simulink model "CVS_LVAD_2021a"  (R2021a)
settings: Solver=ode4  StartTime=0.0  StopTime=end_t  FixedStep=dt_step  RelTol=1e-3
values from neighbouring files (symbols this model uses):
  Cac = 13.7054    [SimMDL_Parameters.m]
  Cbc = 0.25    [SimMDL_Parameters.m]
  Cpa = 1/1.27    (= 0.787401574803)    [SimMDL_Parameters.m]
  Cpv = 1/0.247    (= 4.04858299595)    [SimMDL_Parameters.m]
  Csae = 1/3.02    (= 0.331125827815)    [SimMDL_Parameters.m]
  Csai = 1/7.76    (= 0.128865979381)    [SimMDL_Parameters.m]
  Csve = 1/0.0918    (= 10.8932461874)    [SimMDL_Parameters.m]
  Csvi = 1/0.0989    (= 10.111223458)    [SimMDL_Parameters.m]
  Da0 = 0    [SimMDL_Parameters.m]
  de_gain = 1.5    [SimMDL_Parameters.m]
  delay = 0.5*Tc    (= 0.230769230769)    [SimMDL_Parameters.m]
  deltastar = 0.5    [SimMDL_Parameters.m]
  DElv = 2*(Tc/0.833)    (= 1.10813556192)    [SimMDL_Parameters.m]
  DErv = 2*(Tc/0.833)    (= 1.10813556192)    [SimMDL_Parameters.m]
  Dm0 = 1    [SimMDL_Parameters.m]
  Dp0 = 0    [SimMDL_Parameters.m]
  DRsp = 3*(Tc/0.833)    (= 1.66220334288)    [SimMDL_Parameters.m]
  Dt0 = 1    [SimMDL_Parameters.m]
  dt_step = 1e-3    (= 0.001)    [SimMDL_Parameters.m]
  DTs = 3*(Tc/0.833)    (= 1.66220334288)    [SimMDL_Parameters.m]
  DTv = 0.5    [SimMDL_Parameters.m]
  e_gain = 2    [SimMDL_Parameters.m]
  Elamax = 1.99    [SimMDL_Parameters.m]
  Elamin = 0.733    [SimMDL_Parameters.m]
  Elvmax = 28.4    [SimMDL_Parameters.m]
  Elvmin = 0.550    (= 0.55)    [SimMDL_Parameters.m]
  Eramax = 0.63    [SimMDL_Parameters.m]
  Eramin = 0.317    [SimMDL_Parameters.m]
  Erv_max_sat = 1.2*Ervmax    (= 2.508)    [SimMDL_Parameters.m]
  Erv_max_thres = 0.8*Ervmax    (= 1.672)    [SimMDL_Parameters.m]
  Ervmax = 2.09    [SimMDL_Parameters.m]
  Ervmin = 0.348    [SimMDL_Parameters.m]
  Ga_Elv = 0.012    [SimMDL_Parameters.m]
  Ga_Erv = 0.012    [SimMDL_Parameters.m]
  Ga_Rsp = 0.1    [SimMDL_Parameters.m]
  GaTs = 0.015    [SimMDL_Parameters.m]
  GaTv = 0.028    [SimMDL_Parameters.m]
  Gp_Elv = 0    [SimMDL_Parameters.m]
  Gp_Erv = 0    [SimMDL_Parameters.m]
  Gp_Rsp = 0.33    [SimMDL_Parameters.m]
  GpTs = 0    [SimMDL_Parameters.m]
  GpTv = 0.25    [SimMDL_Parameters.m]
  k_Elv = (Elv_max_sat-Elv_max_thres)/(4*SElvo)    (= 2.84)    [SimMDL_Parameters.m]
  k_Erv = (Erv_max_sat-Erv_max_thres)/(4*SErvo)    (= 0.209)    [SimMDL_Parameters.m]
  k_Rsp = (Rsp_max-Rsp_min)/(4*SRspo)    (= 0.375)    [SimMDL_Parameters.m]
  Kn = max(Kn)    [SimMDL_Parameters.m]
  kT = (T_max-T_min)/(4*STo)    (= 0.035)    [SimMDL_Parameters.m]
  Li = 0.0402    [SimMDL_Parameters.m]
  Lo = 0.0426    [SimMDL_Parameters.m]
  Lsae = 0.0002    [SimMDL_Parameters.m]
  n = length(T)    [SimMDL_Parameters.m]
  pac0 = 0    [SimMDL_Parameters.m]
  pbc0 = 0    [SimMDL_Parameters.m]
  ppa0 = 8.5    [SimMDL_Parameters.m]
  ppv0 = 8    [SimMDL_Parameters.m]
  psae0 = 70    [SimMDL_Parameters.m]
  psai0 = 75    [SimMDL_Parameters.m]
  Psan = 75    [SimMDL_Parameters.m]
  psve0 = 8.7    [SimMDL_Parameters.m]
  psvi0 = 6    [SimMDL_Parameters.m]
  Pth = -3.25    [SimMDL_Parameters.m]
  qi0 = 0    [SimMDL_Parameters.m]
  qo0 = 0    [SimMDL_Parameters.m]
  qsae0 = 10    [SimMDL_Parameters.m]
  Rac = 0.0025    [SimMDL_Parameters.m]
  Ri = 0.4283    [SimMDL_Parameters.m]
  Rm = 0.006    [SimMDL_Parameters.m]
  Ro = 1.2841    [SimMDL_Parameters.m]
  Rpa = 0.006    [SimMDL_Parameters.m]
  Rpp = 0.220    (= 0.22)    [SimMDL_Parameters.m]
  Rpv = 0.006    [SimMDL_Parameters.m]
  Rsae = 0.120    (= 0.12)    [SimMDL_Parameters.m]
  Rsai = 0.016    [SimMDL_Parameters.m]
  Rsp = 2.00    (= 2)    [SimMDL_Parameters.m]
  Rsp_max = 3    [SimMDL_Parameters.m]
  Rsp_min = 1.5    [SimMDL_Parameters.m]
  Rsve = 0.18    [SimMDL_Parameters.m]
  Rsvi = 0.006    [SimMDL_Parameters.m]
  Rtv = 0.006    [SimMDL_Parameters.m]
  t_eject = (Tc*ts_VAD)/dt_step    (= 230.769230769)    [SimMDL_Parameters.m]
  T_max = 0.535    [SimMDL_Parameters.m]
  T_min = 0.395    [SimMDL_Parameters.m]
  Tas = 0.03+0.09*Tc    (= 0.0715384615385)    [SimMDL_Parameters.m]
  Tau_Elv = 1.5    [SimMDL_Parameters.m]
  Tau_Erv = 1.5    [SimMDL_Parameters.m]
  Tau_Rsp = 1.5    [SimMDL_Parameters.m]
  Tau_Ts = 1.8    [SimMDL_Parameters.m]
  Tau_Tv = 0.8    [SimMDL_Parameters.m]
  Tav = 0.01    [SimMDL_Parameters.m]
  Tc = 60/HR    (= 0.461538461538)    [SimMDL_Parameters.m]
  ts_VAD = 0.5    [SimMDL_Parameters.m]
  tune_alpha = x(5)    [SimMDL_Parameters.m]
  tune_gamma = x(3)    [SimMDL_Parameters.m]
  tune_lambda1 = x(1)    [SimMDL_Parameters.m]
  tune_lambda2 = x(2)    [SimMDL_Parameters.m]
  tune_nu = x(4)    [SimMDL_Parameters.m]
  Tvs = 0.16+0.20*Tc    (= 0.252307692308)    [SimMDL_Parameters.m]
  VAD_delay = ts_VAD    (= 0.5)    [SimMDL_Parameters.m]
  vla0 = 11.2524    [SimMDL_Parameters.m]
  Vlau = 1.0    (= 1)    [SimMDL_Parameters.m]
  Vln = 2.3    [SimMDL_Parameters.m]
  vlv0 = 15.6126    [SimMDL_Parameters.m]
  Vlvu = 2.0    (= 2)    [SimMDL_Parameters.m]
  vra0 = 22.36    [SimMDL_Parameters.m]
  Vrau = 1.5    [SimMDL_Parameters.m]
  vrv0 = 26.99    [SimMDL_Parameters.m]
  Vrvu = 3.0    (= 3)    [SimMDL_Parameters.m]
undefined symbols (not defined in the file or in its folder): D_E_max_lv, D_E_max_rv, D_R_svr, D_Ts, D_Tv, f_as_0, f_es_0, f_es_inf, f_es_min, f_ev_0, f_ev_inf, f_max, f_min, G_E_max_lv, G_E_max_rv, G_R_svr, G_Ts, G_Tv, HP_gain, HP_max, HP_min, HP_op, k_es, k_ev, ka, mPsai_op, mPsai_sat, mPsai_thres, passo, pn, Tau_E_max_lv, Tau_E_max_rv, Tau_p, Tau_R_svr, Tau_z
libraries: simulink x6, spsSampleandHoldLib x5, dspmathops x1
(part 2 of 2)

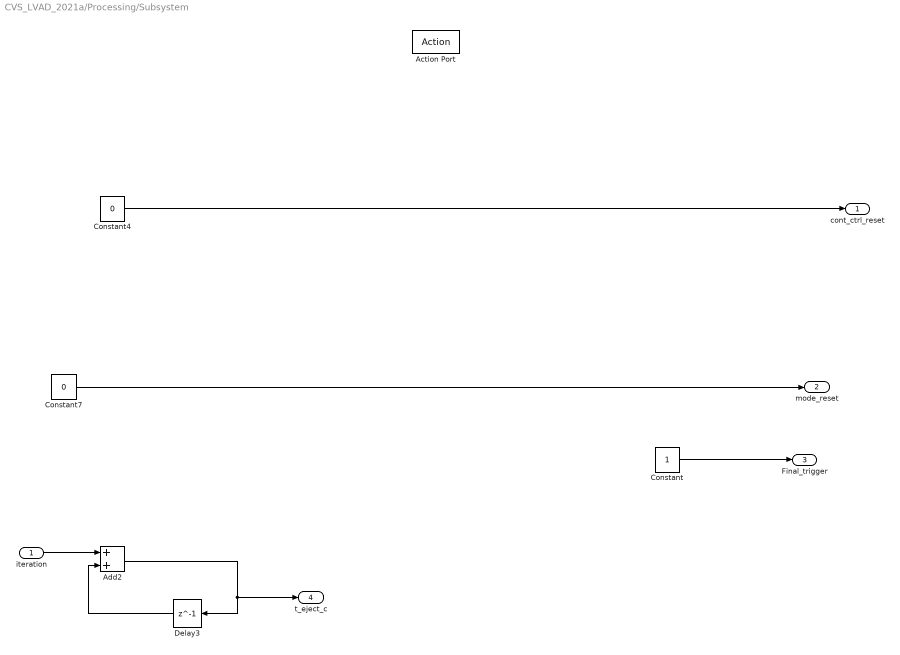
== system CVS_LVAD_2021a/Processing/Subsystem ==
  iteration : Inport
  Action Port : ActionPort  ActionPortLabel=if(u1 > u2)
  Add2 : Sum
  Constant : Constant
  Constant4 : Constant  Value=0
  Constant7 : Constant  Value=0
  Delay3 : Delay  DelayLength=1
  cont_ctrl_reset : Outport
  mode_reset : Outport  Port=2
  Final_trigger : Outport  Port=3
  t_eject_c : Outport  Port=4
  wires:
  Delay3/1 -> Add2/2
  iteration/1 -> Add2/1
  Add2/1 -> t_eject_c/1, Delay3/1
  Constant4/1 -> cont_ctrl_reset/1
  Constant7/1 -> mode_reset/1
  Constant/1 -> Final_trigger/1

== system CVS_LVAD_2021a/Processing/Subsystem1 ==
  Action Port : ActionPort  ActionPortLabel=else
  Constant : Constant  Value=0
  Constant5 : Constant
  Constant8 : Constant
  Cont_ctrl_copy : Outport
  mode_copy : Outport  Port=2
  Final_trigger : Outport  Port=3
  wires:
  Constant8/1 -> mode_copy/1
  Constant5/1 -> Cont_ctrl_copy/1
  Constant/1 -> Final_trigger/1

== system CVS_LVAD_2021a/Processing/Subsystem2 ==
  mode : Inport
  iteration : Inport  Port=2
  t_eject_c : Inport  Port=3
  Action Port : ActionPort  ActionPortLabel=else
  If Action Subsystem : Subsystem  TreatAsAtomicUnit=on
  If2 : If  NumInputs=3  IfExpression=u1 == 1 & u2>=u2  ShowElse=off
  reset : Constant  Value=0
  Out1 : Outport
  Pd_fill : Outport  Port=2
  wires:
  reset/1 -> If Action Subsystem/2(mode_update), If Action Subsystem/1(Pd_fill)
  If2/1 -> If Action Subsystem/Action
  If Action Subsystem/1(Out1) -> Pd_fill/1
  t_eject_c/1 -> If2/3
  mode/1 -> If2/1
  If Action Subsystem/2(Out2) -> Out1/1
  iteration/1 -> If2/2

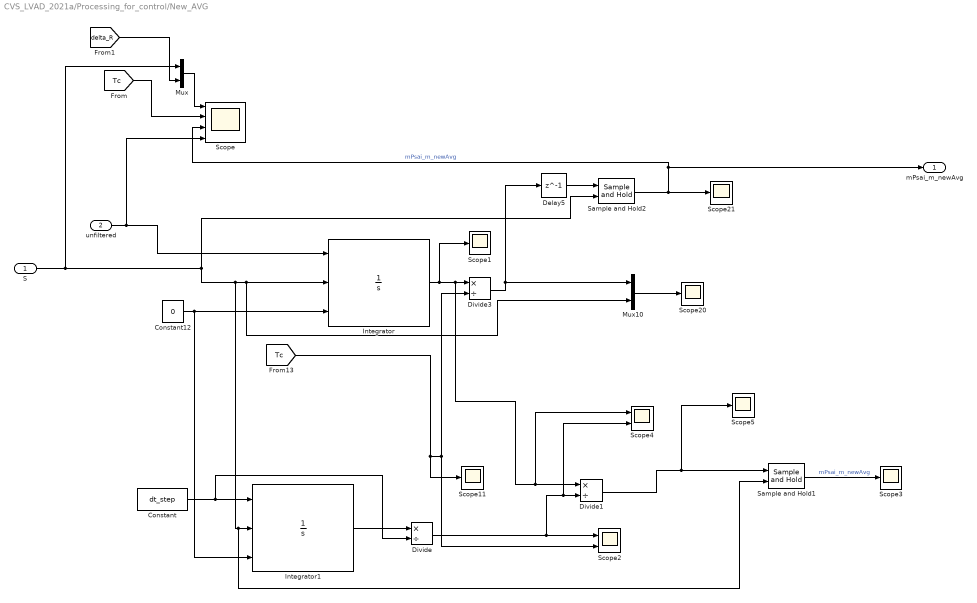
== system CVS_LVAD_2021a/Processing_for_control/New_AVG ==
  S : Inport
  unfiltered : Inport  Port=2
  Constant : Constant  Value=dt_step
  Constant12 : Constant  Value=0
  Delay5 : Delay  DelayLength=1  InitialCondition=psai0
  Divide : Product  Inputs=*/
  Divide1 : Product  Inputs=*/
  Divide3 : Product  Inputs=*/
  Integrator : Integrator  ExternalReset=rising  InitialConditionSource=external
  Integrator1 : Integrator  ExternalReset=rising  InitialConditionSource=external
  Mux : Mux  Inputs=2
  Mux10 : Mux  Inputs=2
  Sample and Hold1 : spsSampleandHoldLib/Sample and Hold  ic=psai0  Ts=dt_step
      settings: SourceProductBaseCode=PS
  Sample and Hold2 : spsSampleandHoldLib/Sample and Hold  ic=psai0  Ts=dt_step
      settings: SourceProductBaseCode=PS
  Scope : Scope  NumInputPorts=4
  Scope{1,3,5,11,20..21} (6 alike) : Scope
  Scope2 : Scope  NumInputPorts=2
  Scope4 : Scope  NumInputPorts=2
  mPsai_m_newAvg : Outport
  wires:
  [Tc] -> Scope2/2, Divide3/2, Scope11/1
  Sample and Hold2/1 -> mPsai_m_newAvg/1, Scope/3, Scope21/1  "mPsai_m_newAvg"
  unfiltered/1 -> Scope/4, Integrator/1
  Delay5/1 -> Sample and Hold2/1
  Mux10/1 -> Scope20/1
  Divide3/1 -> Delay5/1, Mux10/1
  Integrator/1 -> Scope1/1, Scope4/1, Divide1/1, Divide3/1
  Constant12/1 -> Integrator/3, Integrator1/3
  [Tc] -> Scope/2
  [delta_R] -> Mux/2
  Mux/1 -> Scope/1
  Constant/1 -> Divide/2, Integrator1/1
  Integrator1/1 -> Divide/1
  Divide/1 -> Scope4/2, Divide1/2, Scope2/1
  Sample and Hold1/1 -> Scope3/1  "mPsai_m_newAvg"
  Divide1/1 -> Scope5/1, Sample and Hold1/1
  S/1 -> Mux/1, Integrator/2, Mux10/2, Sample and Hold1/2, Integrator1/2, Sample and Hold2/2

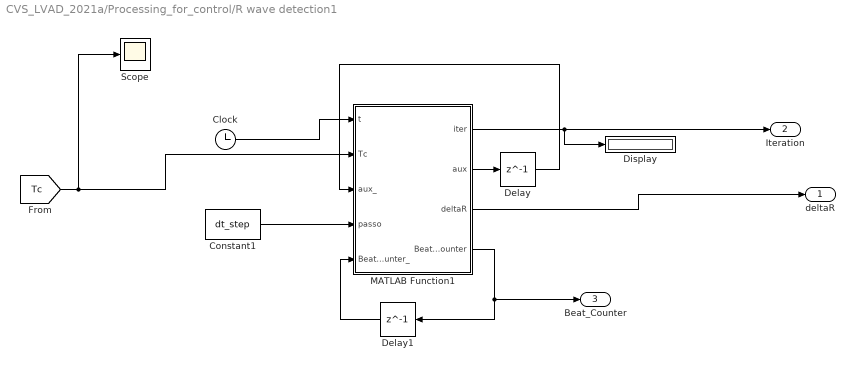
== system CVS_LVAD_2021a/Processing_for_control/R wave detection1 ==
  Clock : Clock
  Constant1 : Constant  Value=dt_step
  Delay : Delay  DelayLength=1
  Delay1 : Delay  DelayLength=1  InitialCondition=0
  Display : Display
  MATLAB Function1 : MATLAB Function  TreatAsAtomicUnit=on
  Scope : Scope
  deltaR : Outport
  Iteration : Outport  Port=2
  Beat_Counter : Outport  Port=3
  wires:
  MATLAB Function1/2(aux) -> Delay/1
  MATLAB Function1/1(iter) -> Display/1, Iteration/1
  Clock/1 -> MATLAB Function1/1(t)
  Constant1/1 -> MATLAB Function1/4(passo)
  MATLAB Function1/3(deltaR) -> deltaR/1
  Delay/1 -> MATLAB Function1/3(aux_)
  MATLAB Function1/4(Beat_Counter) -> Beat_Counter/1, Delay1/1
  Delay1/1 -> MATLAB Function1/5(Beat_Counter_)
  [Tc] -> Scope/1, MATLAB Function1/2(Tc)

== system CVS_LVAD_2021a/Processing_for_control/Subsystem ==
  e(n) : Inport
  e(n-1) : Inport  Port=2
  Gain3 : Gain  Gain=1/dt_step
  Subtract : Sum  Inputs=+-
  de/dt : Outport
  wires:
  Subtract/1 -> Gain3/1
  Gain3/1 -> de/dt/1
  e(n)/1 -> Subtract/1
  e(n-1)/1 -> Subtract/2

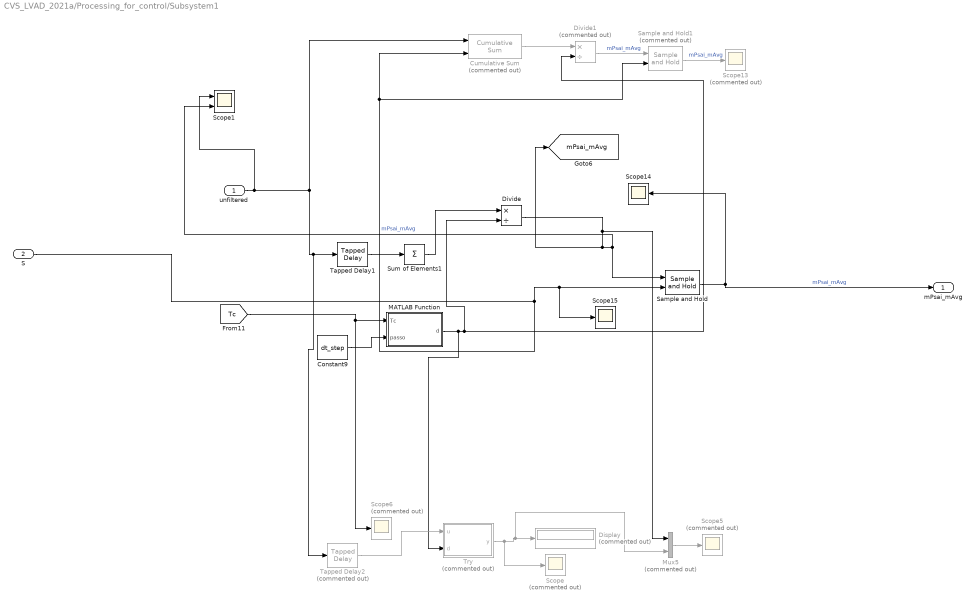
== system CVS_LVAD_2021a/Processing_for_control/Subsystem1 ==
  unfiltered : Inport
  S : Inport  Port=2
  Constant9 : Constant  Value=dt_step
  Cumulative Sum : dspmathops/Cumulative Sum  Commented=on  dim=Channels (running sum)  reset_popup=Non-zero sample  roundingMode=Floor  overflowMode=off  outputDataTypeStr=Inherit: Same as accumulator  outputMin=[]  outputMax=[]  outputLastDataTypeStr=Inherit: Same as accumulator
  Display : Display  Commented=on
  Divide : Product  Inputs=*/
  Divide1 : Product  Commented=on  Inputs=*/
  MATLAB Function : MATLAB Function  TreatAsAtomicUnit=on
  Mux5 : Mux  Commented=on  Inputs=2
  Sample and Hold : spsSampleandHoldLib/Sample and Hold  ic=psai0  Ts=dt_step
      settings: SourceProductBaseCode=PS
  Sample and Hold1 : spsSampleandHoldLib/Sample and Hold  Commented=on  ic=psai0  Ts=passo
      settings: SourceProductBaseCode=PS
  Scope{,5..6,13} (4 alike) : Scope  Commented=on
  Scope1 : Scope  NumInputPorts=2
  Scope14 : Scope
  Scope15 : Scope
  Sum of Elements1 : Sum  Inputs=+
  Tapped Delay1 : simulink/Discrete/Tapped Delay  vinit=psai0  samptime=-1  NumDelays=ceil(Tc/dt_step)  DelayOrder=Oldest  includeCurrent=on
  Tapped Delay2 : simulink/Discrete/Tapped Delay  Commented=on  vinit=psai0  samptime=-1  NumDelays=6000  DelayOrder=Oldest  includeCurrent=on
  Try : MATLAB Function  Commented=on  TreatAsAtomicUnit=on
  mPsai_mAvg : Outport
  tag scope: mPsai_mAvg=global
  wires:
  Sum of Elements1/1 -> Divide/1
  MATLAB Function/1(d) -> Divide1/2, Divide/2, Try/2(d)
  S/1 -> Sample and Hold/2, Scope15/1, Sample and Hold1/2, Cumulative Sum/2
  [Tc] -> MATLAB Function/1(Tc), Scope6/1
  Constant9/1 -> MATLAB Function/2(passo)
  Mux5/1 -> Scope5/1
  unfiltered/1 -> Scope1/1, Tapped Delay2/1, Tapped Delay1/1, Cumulative Sum/1
  Try/1(y) -> Scope/1, Mux5/2, Display/1
  Divide/1 -> Mux5/1, [mPsai_mAvg], Scope1/2, Sample and Hold/1  "mPsai_mAvg"
  Tapped Delay1/1 -> Sum of Elements1/1
  Tapped Delay2/1 -> Try/1(u)
  Sample and Hold/1 -> mPsai_mAvg/1, Scope14/1  "mPsai_mAvg"
  Divide1/1 -> Sample and Hold1/1  "mPsai_mAvg"
  Sample and Hold1/1 -> Scope13/1  "mPsai_mAvg"
  Cumulative Sum/1 -> Divide1/1

== system CVS_LVAD_2021a/Processing/Subsystem2/If Action Subsystem ==
  Pd_fill : Inport
  mode_update : Inport  Port=2
  Action Port : ActionPort  ActionPortLabel=if(u1 == 1 & u2>=u2)
  Out1 : Outport
  Out2 : Outport  Port=2
  wires:
  Pd_fill/1 -> Out1/1
  mode_update/1 -> Out2/1

== matlab function CVS_LVAD_2021a/Baroreflex Model_Liu/MATLAB Function3 ==
  data: G_E_max_rv input; sigma_E_max_rv output; f_es_min input; f_es input
function sigma_E_max_rv = fcn(G_E_max_rv,f_es_min,f_es)

if(f_es>=f_es_min)
    sigma_E_max_rv = G_E_max_rv*log(f_es-f_es_min+1);
else
    sigma_E_max_rv = 0;
end

== matlab function CVS_LVAD_2021a/Baroreflex Model_Liu/MATLAB Function4 ==
  data: G_Ts input; sigma_Ts output; f_es_min input; f_es input
function sigma_Ts = fcn(G_Ts,f_es_min,f_es)

if(f_es>=f_es_min)
    sigma_Ts = G_Ts*log(f_es-f_es_min+1);
else
    sigma_Ts = 0;
end

== matlab function CVS_LVAD_2021a/Heart+LVAD1/MATLAB Function ==
  data: Tas input; Kn output; Tav input; Tvs input; Tc input; n input; iter input
function Kn = fcn(Tas,Tav,Tvs,Tc,n,iter)
Kn_=zeros(1,n);
for k = 1:n
   j = mod(iter, Tc);
   Kn_(k) = ((j-(Tas + Tav))/Tvs)*sin((pi*(j-(Tas + Tav))/Tvs));
end
Kn = max(Kn_);

== matlab function CVS_LVAD_2021a/Controller/MATLAB Function1 ==
  data: PID input; u output; Dual input; SM input; sw input
function u = fcn(PID,Dual,SM,sw)

if(sw==0)
    u=PID;
elseif(sw==1)
    u=SM;
else
    u=Dual;
end

== matlab function CVS_LVAD_2021a/Processing_for_control/Subsystem1/MATLAB Function ==
  data: Tc input; d output; passo input
function d = fcn(Tc,passo)
%#codegen
d=(ceil(Tc/passo));

== matlab function CVS_LVAD_2021a/Processing_for_control/Subsystem1/Try ==
  data: u input; y output; d input
function y = fcn(u,d)

sum=0;
for i= (5000-d+1):5000
    sum=sum+u(i);
end
y=sum/d;

== matlab function CVS_LVAD_2021a/Ursino Model/MATLAB Function1 ==
  data: t input; HP output; HP_baro input; HP_Prev input
function HP = fcn(t,HP_baro,HP_Prev)

if(t>0)
    if(mod(t,5)==0)
        HP=HP_baro;
    else
        HP=HP_Prev;
    end
else
    HP=HP_Prev;
end

== matlab function CVS_LVAD_2021a/Controller/Cordeiro's _Controller ==
  data: Pe_n_1 input; Pe output; Pe_n_2 input; Pe_n_3 input; e_n input; e_n_1 input; e_n_2 input; e_n_3 input
function Pe = fcn(Pe_n_1,Pe_n_2, Pe_n_3,e_n, e_n_1,  e_n_2, e_n_3)

num = [1.0000    2.3082   -0.1752    0.0017];
b0 =  num(1);
b1 =  num(2);
b2 =  num(3);
b3 =  num(4);

den = [1.0000   -0.4633   -0.9876    0.4509];
a0 =  den(1);
a1 =  den(2);
a2 =  den(3);
a3 =  den(4);
%Pe = (-a1/a0)*Pe(ii-1) + (-a2/a0)*Pe(ii-2) + (-a3/a0)*Pe(ii-3)...
                         %  + (b0/a0)*e(ii) + (b1/a0)*e(ii-1) + (b2/a0)*e(ii-2) + (b3/a0)*e(ii-3);
Pe = (-a1/a0)*Pe_n_1 + (-a2/a0)*Pe_n_2 + (-a3/a0)*Pe_n_3 + (b0/a0)*e_n + (b1/a0)*e_n_1 + (b2/a0)*e_n_2 + (b3/a0)*e_n_3;

== matlab function CVS_LVAD_2021a/Processing_for_control/Fig7_Cordeiro2020 ==
  data: Beats_c input; mPsai_ref output
function mPsai_ref = fcn(Beats_c)

mPsai_ref=75;
if (Beats_c >= 25) && (Beats_c < 70)
    mPsai_ref = 85;
elseif (Beats_c >=70)
    mPsai_ref = 80;

end

== matlab function CVS_LVAD_2021a/Ursino Model/Sigmoid_Rsp ==
  data: Rsp_min input; sigma_Rsp output; Rsp_max input; k_Rsp input; x_Rsp input
function sigma_Rsp = fcn(Rsp_min,Rsp_max,k_Rsp,x_Rsp)


num=Rsp_min+Rsp_max*exp(-x_Rsp/k_Rsp);
den=1+exp(-x_Rsp/k_Rsp);
sigma_Rsp = num/den;

== matlab function CVS_LVAD_2021a/Ursino Model/Sigmoid_T ==
  data: T_min input; T output; T_max input; kT input; xT input
function T = fcn(T_min,T_max,kT,xT)

num=T_min+T_max*exp(xT/kT);
den=1+exp(xT/kT);
T=num/den;

== matlab function CVS_LVAD_2021a/Ursino Model/Sigmoid_Rsp1 ==
  data: Erv_min input; sigma_Erv output; Erv_max input; k_Erv input; x_Erv input
function sigma_Erv = fcn(Erv_min,Erv_max,k_Erv,x_Erv)


num=Erv_min+Erv_max*exp(-x_Erv/k_Erv);
den=1+exp(-x_Erv/k_Erv);
sigma_Erv = num/den;

== matlab function CVS_LVAD_2021a/Ursino Model/MATLAB Function ==
  data: Y_min input; Y output; Y_max input; X_thres input; X_sat input; X0 input; Y0 input; X input; gain input
function Y = fcn(Y_min,Y_max,X_thres,X_sat,X0,Y0,X,gain)

%X0 and Y0 are redundant
if(X<=X_thres)
    Y=Y_min;
elseif(X>=X_sat)
    Y=Y_max;
else
    Y=Y0+gain*(X-X0);
end

== matlab function CVS_LVAD_2021a/Ursino Model/Sigmoid_Rsp2 ==
  data: Elv_min input; sigma_Elv output; Elv_max input; k_Elv input; x_Elv input
function sigma_Elv = fcn(Elv_min,Elv_max,k_Elv,x_Elv)


num=Elv_min+Elv_max*exp(-x_Elv/k_Elv);
den=1+exp(-x_Elv/k_Elv);
sigma_Elv = num/den;

== matlab function CVS_LVAD_2021a/Processing_for_control/Fig7_Cordeiro1 ==
  data: t input; mPsai_ref output
function mPsai_ref = fcn(t)

mPsai_ref=75;
if (t >= 20) && (t < 25)
    mPsai_ref = 75+(t-20)*(85-75)/(25-20);
elseif (t >=25 && t<40)
    mPsai_ref= 85;
elseif (t >=40 && t<45)
    mPsai_ref = 85+(t-40)*(80-85)/(45-40);
elseif(t>=45)
    mPsai_ref=80;
end

== matlab function CVS_LVAD_2021a/Controller/MATLAB Function ==
  data: e input; s output
function s = fcn(e)

if(abs(e)<=3)
    s=1;
else
    s=0;
end

== matlab function CVS_LVAD_2021a/Baroreflex Model_Liu/MATLAB Function ==
  data: f_min input; f_as output; f_max input; pn input; ka input; p input
function f_as = fcn(f_min,f_max,pn,ka,p)

exp_comp = exp((p-pn)/ka);
f_as = (f_min+f_max*exp_comp)/(1+exp_comp);

== matlab function CVS_LVAD_2021a/Controller/SMC_CONTROLLER /MATLAB Function ==
  data: e input; sl_man output; sign_s output; u output; e_dot input; lambda1 input; lambda2 input; gamma input; nu input; alpha input
function [sl_man,sign_s, u]  = fcn(e,e_dot, lambda1,lambda2,gamma,nu,alpha)


%% CONTROLLER-4: Semi-Hyperbolic Tangent SMC
% lambda1 = 2; nu = 10; alpha = 1; gamma = 12;
% lambda2 = 1;
sl_man = lambda1*e+lambda2*e_dot;
sign_s = sign(sl_man);
if sl_man>nu
    h = 1;
elseif -nu<=sl_man && sl_man<=nu
    h = tanh(alpha*(sl_man/nu))/tanh(alpha);
else
    h = -1;
end
u = 1*gamma*h;

== matlab function CVS_LVAD_2021a/Processing_for_control/Hold ==
  data: delta_lvad input; Pd output; Pe input; mode_ input; mode output; Pd_ input; t_eject input; t_eject_c_ input; t_eject_c output; iteration input; cont_ctrl_ input; cont_ctrl output; deltastar input; Tc input; passo input; delta_lvad_ output; trig output; pe_ input; pe output
function [Pd,mode,t_eject_c,cont_ctrl,delta_lvad_,trig,pe] = fcn(delta_lvad,Pe,mode_,Pd_,t_eject,t_eject_c_,iteration,cont_ctrl_,deltastar,Tc,passo,pe_)
pe=pe_;
Pd=Pd_;
mode=mode_;
t_eject_c=t_eject_c_;
cont_ctrl = cont_ctrl_;
delta_lvad_=delta_lvad;
trig=0;
if(mode==0)
    if(delta_lvad==1)
        cont_ctrl=cont_ctrl+1;
        if(cont_ctrl > deltastar*Tc/passo)
            delta_lvad_=0;
            cont_ctrl=0;
            mode=1;
            Pd = Pe;
            pe = Pe;
            t_eject_c = iteration + t_eject;
            trig = 1;
        end
    end
else
    if(iteration >=t_eject_c)
        Pd=0;
        mode=0;
    end
end

== matlab function CVS_LVAD_2021a/Processing_for_control/Psai_Train_Reference_gen1 ==
  data: Beats_c input; mPsai_ref output
function mPsai_ref = fcn(Beats_c)

mPsai_ref=80;
if (Beats_c >= 20) && (Beats_c < 30)
    mPsai_ref = 85;
elseif (Beats_c >= 30) && (Beats_c < 50)
    mPsai_ref = 80;
elseif (Beats_c >= 50) && (Beats_c < 70)
    mPsai_ref = 90;
elseif Beats_c >= 70
    mPsai_ref = 80;
end

== matlab function CVS_LVAD_2021a/Processing_for_control/R wave detection1/MATLAB Function1 ==
  data: t input; Tc input; iter output; aux_ input; passo input; aux output; deltaR output; Beat_Counter_ input; Beat_Counter output
function [iter,aux,deltaR,Beat_Counter]= fcn(t,Tc,aux_,passo,Beat_Counter_)

Beat_Counter=Beat_Counter_;
if(t>=aux_*Tc)
    deltaR=1;
    Beat_Counter=Beat_Counter+1;
    aux=aux_+1;
else
    deltaR=0;
    aux=aux_;
end
iter=t/passo+1;

== matlab function CVS_LVAD_2021a/Processing_for_control/Trigger Engine ==
  data: deltaR input; delta_lvad output; delay input; iter input; trig_iter input; trig_iter_ output; passo input; delta_lvad_ input
function [delta_lvad,trig_iter_] = fcn(deltaR,delay,iter,trig_iter,passo,delta_lvad_)

trig_iter_=trig_iter;
delta_lvad=delta_lvad_;
if(iter>trig_iter && trig_iter_>0)  %trig_iter is when lvad must be triggered.
    delta_lvad=1;
    trig_iter_=0;
else
    if(deltaR>0)
        trig_iter_= iter + fix(delay/passo);
    end
end

== matlab function CVS_LVAD_2021a/Heart+LVAD1/Ela ==
  data: Time input; Ela output; Elamin input; Elamax input; Tc input; avt output
function [Ela,avt] = fcn(Time,Elamin,Elamax,Tc)
t=mod(Time,Tc);
Tas = 0.03+0.09*Tc;
% Emin Emax declared seperately

if(t>=0 && t<Tas)
    avt = sin(pi*t/Tas);
else
    avt=0;
end
Ela = (Elamin+avt*(Elamax-Elamin));
%C=1/Et;

== matlab function CVS_LVAD_2021a/Heart+LVAD1/Elv ==
  data: Time input; Elv output; Elvmin input; Elvmax input; Tc input; Kn input; avt output
function [Elv,avt] = fcn(Time,Elvmin,Elvmax,Tc,Kn)
t=mod(Time,Tc);
Tas = 0.03+0.09*Tc;
Tvs = 0.16+0.20*Tc;
Tav=0.01;
Tavi= Tas+Tav;
Tavf=Tas+Tav+Tvs;
% Kn Find from simulating separately
% Emin Emax declared seperately

if(t>= Tavi && t<Tavf)
    c1 = (t-(Tas+Tav))/(Tvs);
    avt = (c1/Kn)*sin(pi*c1);
else
    avt=0;
end
Elv = (Elvmin+avt*(Elvmax-Elvmin));
%C=1/Et;

== matlab function CVS_LVAD_2021a/Heart+LVAD1/Era ==
  data: Time input; Era output; Eramin input; Eramax input; Tc input; avt output
function [Era,avt] = fcn(Time,Eramin,Eramax,Tc)
t=mod(Time,Tc);
Tas = 0.03+0.09*Tc;
% Emin Emax declared seperately

if(t>=0 && t<Tas)
    avt = sin(pi*t/Tas);
else
    avt=0;
end
Era = (Eramin+avt*(Eramax-Eramin));
%C=1/Et;

== matlab function CVS_LVAD_2021a/Processing/Trigger Engine ==
  data: deltaR input; delta_lvad output; delay input; iter input; trig_iter input; trig_iter_ output; passo input; delta_lvad_ input
function [delta_lvad,trig_iter_] = fcn(deltaR,delay,iter,trig_iter,passo,delta_lvad_)

trig_iter_=trig_iter;
delta_lvad=delta_lvad_;
if(iter>trig_iter && trig_iter_>0)  %trig_iter is when lvad must be triggered.
    delta_lvad=1;
    trig_iter_=0;
else
    if(deltaR>0)
        trig_iter_= iter + fix(delay/passo);
    end
end

== matlab function CVS_LVAD_2021a/Heart+LVAD1/Erv ==
  data: Time input; Erv output; Ervmin input; Ervmax input; Tc input; Kn input; avt output
function [Erv,avt] = fcn(Time,Ervmin,Ervmax,Tc,Kn)
t=mod(Time,Tc);
Tas = 0.03+0.09*Tc;
Tvs = 0.16+0.20*Tc;
Tav=0.01;
Tavi= Tas+Tav;
Tavf=Tas+Tav+Tvs;
% Kn Find from simulating separately
% Emin Emax declared seperately

if(t>= Tavi && t<Tavf)
    c1 = (t-(Tas+Tav))/(Tvs);
    avt = (c1/Kn)*sin(pi*c1);
else
    avt=0;
end
Erv = (Ervmin+avt*(Ervmax-Ervmin));
%C=1/Et;

== matlab function CVS_LVAD_2021a/Heart+LVAD1/Heart_Valves ==
  data: Pra input; Dt output; Prv input; Pla input; Plv input; Ppa input; Dp output; Dm output; Da output; Pao input
function [Dt,Dp,Dm,Da] = fcn(Pra,Prv,Pla,Plv,Ppa,Pao)

if ((Pla - Plv) > 0)
    Dm = 1;
else
    Dm = 0;
end

if ((Plv - Pao) > 0)
    Da = 1;
else
    Da = 0;
end

if ((Pra - Prv) > 0)
    Dt = 1;
else
    Dt = 0;
end

if ((Prv - Ppa) > 0)
    Dp = 1;
else
    Dp = 0;
end

== matlab function CVS_LVAD_2021a/Heart+LVAD1/Klin ==
  data: Ppv_Pla input; Klin output
function Klin = fcn(Ppv_Pla)

if(Ppv_Pla>=0)
    Klin=1;
else
    Klin=100;
end

== matlab function CVS_LVAD_2021a/Heart+LVAD1/Lvad_Valves ==
  data: Pbc input; Di output; Do output; Pac input; Plv input; Pao input
function [Di,Do] = fcn(Pbc,Pac,Plv,Pao)

if (Plv - (Pac+Pbc)) > 0
    Di = 1;
else
    Di = 0;
end

if ((Pac+Pbc) - Pao) > 0
    Do = 1;
else
    Do=0;
end

== matlab function CVS_LVAD_2021a/Heart+LVAD1/Pao ==
  data: Psai input; Pao_ output; qsai input; Rsai input
function Pao_ = fcn(Psai,qsai,Rsai)

Pao_ = Psai+Rsai*qsai;

== matlab function CVS_LVAD_2021a/Heart+LVAD1/Pla ==
  data: Ela input; Pla output; Vla input; Vlau input
function Pla = fcn(Ela,Vla,Vlau)

Pla = Ela*(Vla-Vlau);

== matlab function CVS_LVAD_2021a/Heart+LVAD1/Plv ==
  data: Elv input; Plv output; Vlv input; Vlvu input
function Plv = fcn(Elv,Vlv,Vlvu)

Plv = Elv*(Vlv-Vlvu);

== matlab function CVS_LVAD_2021a/Heart+LVAD1/Pra = Ela*(Vra - Vrau) ==
  data: Era input; Pra output; Vra input; Vrau input
function Pra = fcn(Era,Vra,Vrau)

Pra = Era*(Vra-Vrau);

== matlab function CVS_LVAD_2021a/Heart+LVAD1/Prv = Erv*(Vrv - Vrvu) ==
  data: Erv input; Prv output; Vrv input; Vrvu input
function Prv = fcn(Erv,Vrv,Vrvu)

Prv = Erv*(Vrv-Vrvu);

== matlab function CVS_LVAD_2021a/Heart+LVAD1/dPac//dt = (-1//(Rac*Cac))*Pac + (1//(Rac*Cac))*Pd ==
  data: Pac input; dPac output; Pd input; Rac input; Cac input
function dPac = fcn(Pac,Pd,Rac,Cac)

dPac = (-Pac+Pd)/(Rac*Cac);

== matlab function CVS_LVAD_2021a/Heart+LVAD1/dPbc//dt = (1//Cbc)*qi - (1//Cbc)*qo ==
  data: qi input; dPbc output; qo input; Cbc input
function dPbc = fcn(qi,qo,Cbc)

dPbc = (qi-qo)/Cbc;

== matlab function CVS_LVAD_2021a/Heart+LVAD1/dPpa//dt  = (qpa - qpp)//Cpa ==
  data: qpa input; dPpa output; qpp input; Cpa input
function dPpa = fcn(qpa,qpp,Cpa)

dPpa = (qpa-qpp)/Cpa;

== matlab function CVS_LVAD_2021a/Heart+LVAD1/dPpv//dt = (qpp - qla)//Cpv ==
  data: qpp input; dPpv output; qla input; Cpv input
function dPpv = fcn(qpp,qla,Cpv)

dPpv = (qpp-qla)/Cpv;

== matlab function CVS_LVAD_2021a/Heart+LVAD1/dPsae//dt  = (qsae - qsp)//Csae ==
  data: qsae input; dPsae output; qsp input; Csae input; Vusae_dot input
function dPsae = fcn(qsae,qsp,Csae,Vusae_dot)

dPsae = (qsae-qsp-Vusae_dot)/Csae;

== matlab function CVS_LVAD_2021a/Baroreflex Model_Liu/Sympathetic ==
  data: f_es_inf input; f_es output; f_es_0 input; k_es input; f_as input
function f_es = fcn(f_es_inf,f_es_0,k_es,f_as)

f_es = f_es_inf+(f_es_0-f_es_inf)*exp(-k_es*f_as);

== matlab function CVS_LVAD_2021a/Heart+LVAD1/dPsai//dt  = (qsai + qo - qsae)//Csai ==
  data: qsai input; dPsai output; qo input; qsae input; Csai input
function dPsai = fcn(qsai,qo,qsae,Csai)

dPsai = (qsai+qo-qsae)/Csai;

== matlab function CVS_LVAD_2021a/Heart+LVAD1/dPsve//dt  = (qsp - qsve)//Csve ==
  data: qsp input; Psve output; qsve input; Csve input; Vusve_dot input
function Psve = fcn(qsp,qsve,Csve,Vusve_dot)

Psve = (qsp-qsve-Vusve_dot)/Csve;

== matlab function CVS_LVAD_2021a/Heart+LVAD1/dPsvi//dt  = (qsve - qra)//Csvi ==
  data: qsve input; dPsvi output; qra input; Csvi input
function dPsvi = fcn(qsve,qra,Csvi)

dPsvi = (qsve-qra)/Csvi;

== matlab function CVS_LVAD_2021a/Heart+LVAD1/dVla//dt  = qla - qmv ==
  data: qla input; dVla output; qmv input
function dVla = fcn(qla,qmv)

dVla = qla-qmv;

== matlab function CVS_LVAD_2021a/Heart+LVAD1/dVlv//dt  = qmv - qsai - qi ==
  data: qmv input; dVlv output; qsai input; qi input
function dVlv = fcn(qmv,qsai,qi)

dVlv = qmv-qsai-qi;

== matlab function CVS_LVAD_2021a/Heart+LVAD1/dqi//dt = -(Ri//Li)*qi - Di*(1//Li)*(Pbc+Pac) + Di*(1//Li)*plv ==
  data: qi input; dqi output; Pbc input; Pac input; Plv input; Ri input; Li input; Di input
function dqi = fcn(qi,Pbc,Pac,Plv,Ri,Li,Di)

dqi = (-Ri*qi-(Di*(Pac+Pbc))+Di*Plv)/Li;

== matlab function CVS_LVAD_2021a/Heart+LVAD1/dqo//dt = -(Ro//Lo)*qo + Do*(1//Lo)*(Pac+Pbc) - Do*(1//Lo)*pao ==
  data: qo input; dqo output; Pbc input; Pac input; Pao input; Ro input; Lo input; Do input
function dqo = fcn(qo,Pbc,Pac,Pao,Ro,Lo,Do)

dqo = (-Ro*qo+(Do*(Pac+Pbc))-Do*Pao)/Lo;

== matlab function CVS_LVAD_2021a/Heart+LVAD1/dqsae//dt = (psai + Pth - psae - Rsae*qsae)//Lsae ==
  data: Psai input; dqsae output; Pth input; Psae input; qsae input; Rsae input; Lsae input
function dqsae = fcn(Psai,Pth,Psae,qsae,Rsae,Lsae)

dqsae = (Psai + Pth - Psae - Rsae*qsae)/Lsae;

== matlab function CVS_LVAD_2021a/Heart+LVAD1/qmv  = Dm*(Pla -  Plv)//Rmv ==
  data: Dm input; qmv output; Pla input; Plv input; Rmv input
function qmv = fcn(Dm,Pla,Plv,Rmv)

qmv = Dm*(Pla-Plv)/Rmv;

== matlab function CVS_LVAD_2021a/Processing/R wave detection1/MATLAB Function1 ==
  data: t input; HR input; iter output; aux_ input; passo input; aux output; deltaR output; Beat_Counter_ input; Beat_Counter output
function [iter,aux,deltaR,Beat_Counter]= fcn(t,HR,aux_,passo,Beat_Counter_)

Beat_Counter=Beat_Counter_;
if(t>=aux_*60/HR)
    deltaR=1;
    Beat_Counter=Beat_Counter+1;
    aux=aux_+1;
else
    deltaR=0;
    aux=aux_;
end
iter=t/passo+1;

== matlab function CVS_LVAD_2021a/Heart+LVAD1/qpa ==
  data: Prv input; qpa output; Ppa input; Rpa input; Dp input
function qpa= fcn(Prv,Ppa,Rpa,Dp)

qpa = Dp*(Prv-Ppa)/Rpa;

== matlab function CVS_LVAD_2021a/Heart+LVAD1/qpp ==
  data: Ppa input; qpp output; Ppv input; Rpp input
function qpp = fcn(Ppa,Ppv,Rpp)

qpp = (Ppa-Ppv)/Rpp;

== matlab function CVS_LVAD_2021a/Heart+LVAD1/qra ==
  data: Psvi input; qra output; Pra input; Rsvi input
function qra = fcn(Psvi,Pra,Rsvi)


if((Psvi - Pra) >= 0)
    qra= (Psvi-Pra)/(Rsvi);
else
    qra= (Psvi-Pra)/(Rsvi*100);
end

== matlab function CVS_LVAD_2021a/Heart+LVAD1/qsai ==
  data: Plv input; qsai output; Psai input; Da input; qo input; Rsai input
function qsai = fcn(Plv,Psai,Da,qo,Rsai)

if(Da==1)
    qsai = (Plv - Psai)/Rsai;
else
    qsai = qo;
end

== matlab function CVS_LVAD_2021a/Heart+LVAD1/qsp ==
  data: Psae input; Psve input; qsp output; Rsp input
function qsp = fcn(Psae,Psve,Rsp)

qsp = (Psae-Psve)/Rsp;

== matlab function CVS_LVAD_2021a/Heart+LVAD1/qsve ==
  data: Psve input; qsve output; Psvi input; Pth input; Rsve input
function qsve = fcn(Psve,Psvi,Pth,Rsve)

qsve = (Psve-(Psvi+Pth))/Rsve;

== matlab function CVS_LVAD_2021a/Heart+LVAD1/qtv ==
  data: Pra input; qtv output; Prv input; Rtv input; Dt input
function qtv = fcn(Pra,Prv,Rtv,Dt)

qtv = Dt*(Pra-Prv)/Rtv;

== matlab function CVS_LVAD_2021a/Baroreflex Model_Liu/Vagus ==
  data: f_ev_0 input; f_ev output; f_ev_inf input; f_as_0 input; k_ev input; f_as input
function f_ev = fcn(f_ev_0,f_ev_inf,f_as_0,k_ev,f_as)

exp_comp = exp((f_as-f_as_0)/k_ev);
f_ev = (f_ev_0+f_ev_inf*exp_comp)/(1+exp_comp);

== matlab function CVS_LVAD_2021a/Baroreflex Model_Liu/MATLAB Function1 ==
  data: G_R_svr input; sigma_Ts output; f_es_min input; f_es input
function sigma_Ts = fcn(G_R_svr,f_es_min,f_es)

if(f_es>=f_es_min)
    sigma_Ts = G_R_svr*log(f_es-f_es_min+1);
else
    sigma_Ts = 0;
end

== matlab function CVS_LVAD_2021a/Baroreflex Model_Liu/MATLAB Function2 ==
  data: G_E_max_lv input; sigma_E_max_lv output; f_es_min input; f_es input
function sigma_E_max_lv = fcn(G_E_max_lv,f_es_min,f_es)

if(f_es>=f_es_min)
    sigma_E_max_lv = G_E_max_lv*log(f_es-f_es_min+1);
else
    sigma_E_max_lv = 0;
end
